simulink model "Reloadable_FIR"  (R2020a)
settings: Solver=VariableStepDiscrete  StartTime=0.0  StopTime=60  MaxStep=1  RelTol=1e-3  EnableMultiTasking=on
libraries: xbsIndex_r4 x15, dspsrcs4 x3, xbsCopyrightNotice_r4 x1
settings Model: Creator=arvinds  LastModifiedBy=viswanad
settings DataIOCC: LimitDataPoints=on  SaveFormat=Array  SignalLoggingSaveFormat=ModelDataLogs  ReturnWorkspaceOutputs=off
settings OptimizationCC: DefaultParameterBehavior=Inlined  ExpressionDepthLimit=2147483647  InitFltsAndDblsToZero=on  LifeSpan=inf
settings DebuggingCC: SaveWithParameterizedLinksMsg=none  UnderspecifiedInitializationDetection=Classic  MergeDetectMultiDrivingBlocksExec=none  SignalResolutionControl=TryResolveAllWithWarning  SolverPrmCheckMsg=warning  MultiTaskDSMMsg=warning  MultiTaskCondExecSysMsg=none  FcnCallInpInsideContextMsg=warning  AllowSymbolicDim=off  StateNameClashWarn=warning  SFUnexpectedBacktrackingDiag=warning  SFNoUnconditionalDefaultTransitionDiag=warning  SFExecutionAtInitializationDiag=none  ArithmeticOperatorsInVariantConditions=warning
settings HardwareCC: ProdBitPerPointer=32  ProdBitPerSizeT=32  ProdBitPerPtrDiffT=32  ProdLargestAtomicFloat=None  ProdIntDivRoundTo=Undefined  ProdEndianess=Unspecified  ProdWordSize=32  ProdHWDeviceType=32-bit Generic
settings ModelReferenceCC: PropagateSignalLabelsOutOfModel=off
settings SFSimCC: SimUseLocalCustomCode=off  CustomCodeUndefinedFunction=UseInterfaceOnly
settings RTWCC: RTWUseLocalCustomCode=off
settings CodeAppCC: StateflowObjectComments=on
settings GRTTargetCC: TargetFcnLib=ansi_tfl_tmw.mat  TargetLangStandard=C89/C90 (ANSI)  CombineOutputUpdateFcns=off  GRTInterface=on
settings ConfigComp: CovMetricSettings=dw  CovSaveCumulativeToWorkspaceVar=on  CovSaveSingleToWorkspaceVar=on  CovExternalEMLEnable=off

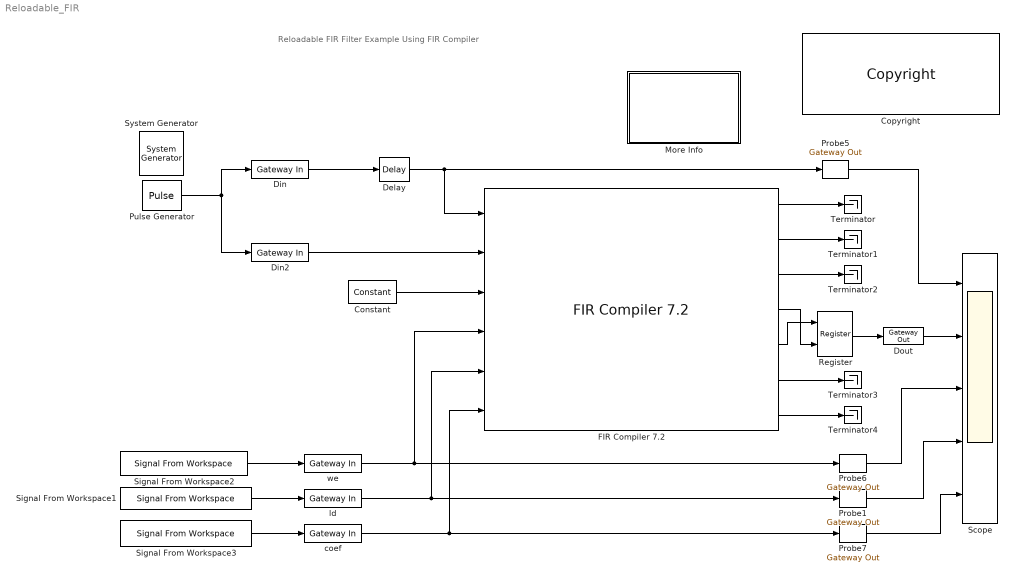
== system Reloadable_FIR ==
  note: Reloadable FIR Filter Example Using FIR Compiler
  " System Generator" : xbsIndex_r4/ System Generator  Tag=genX  xilinxfamily=kintex7  part=xc7k325t  speed=-3  package=fbg676  synthesis_tool=Vivado  clock_wrapper=Clock Enables  directory=./netlist  proj_type=Vivado  Synth_file=Vivado Synthesis Defaults  Impl_file=Vivado Implementation Defaults  testbench=off  simulink_period=1  sysclk_period=10  dcm_input_clock_period=10  incr_netlist=off  trim_vbits=Everywhere in SubSystem  dbl_ovrd=According to Block Masks  core_generation=According to Block Masks  run_coregen=off  deprecated_control=off  eval_field=0  block_type=sysgen
  Constant : xbsIndex_r4/Constant  const=0  gui_display_data_type=Fixed-point  arith_type=Unsigned  n_bits=8  bin_pt=0  preci_type=Single  exp_width=8  frac_width=24  explicit_period=off  period=1  equ=P=C  opselect=C  inp2=PCIN>>17  opr=+  inp1=P  carry=CIN  dbl_ovrd=off  block_type=constant
  Copyright : xbsCopyrightNotice_r4/Copyright  copyrighttext="Copyright (c) 2021  by  Xilinx, Inc. All rights reserved.<br><br>This file contains proprietary, confidential information of Xilinx, Inc., is distributed under license from Xilinx, Inc., and may be used, copied and/or disclosed only pursuant to the terms of a valid license agreement with Xilinx, Inc. Xilinx hereby grants you a license to use this file solely for design, simulation, implementation and creation of design files limited to Xilinx devices or technologies. Use with non-Xilinx devices or technologies is expressly prohibited and immediately terminates your license unless covered by a separate agreement.<br><br>Xilinx is providing this design, code, or information \"as-is\" solely for use in developing programs and solutions for Xilinx devices, with no obligation on the part of Xilinx to provide support. By providing this design, code, or information as one possible implementation of this feature, application or standard, Xilinx is making no representation that this implementation is free from any claims of infringement. You are responsible for obtaining any rights you may require for your implementation. Xilinx expressly disclaims any warranty whatsoever with respect to the adequacy of the implementation, including but not limited to any warranties or representations that this implementation is free from claims of infringement, implied warranties of merchantability or fitness for a particular purpose.<br><br>Xilinx products are not intended for use in life support appliances, devices, or systems. Use in such applications is expressly prohibited.<br><br>Any modifications that are made to the Source Code are done at the user's sole risk and will be unsupported.<br><br>This copyright and support notice must be retained as part of this text at all times. (c) Copyright 1995-2021 Xilinx, Inc. All rights reserved."  block_type=copyright
  Delay : xbsIndex_r4/Delay  rst=off  infoeditControl=Selection of Reset will increase slice count due to use of real FFs and instead of SRLs  en=off  latency=1  reg_retiming=off  dbl_ovrd=off  block_type=delay
  Din : xbsIndex_r4/Gateway In  gui_display_data_type=Fixed-point  arith_type="Signed  (2's comp)"  n_bits=16  bin_pt=0  preci_type=Single  exp_width=8  frac_width=24  rows=1  columns=1  quantization="Round  (unbiased: +/- Inf)"  overflow=Saturate  period=1  UseAsADC=off  ADCChannel='1'  interface=None  automatic_assignment=on  address_offset=hex2dec('00')  intf_name=''  intf_description=''  default_value=0  timing_constraint=None  locs_specified=off  LOCs={}  io_standard={}  inherit_from_input=off  hdl_port=on  dbl_ovrd=off  block_type=gatewayin
  Din2 : xbsIndex_r4/Gateway In  gui_display_data_type=Boolean  arith_type=Boolean  n_bits=8  bin_pt=0  preci_type=Single  exp_width=8  frac_width=24  rows=1  columns=1  quantization="Round  (unbiased: +/- Inf)"  overflow=Saturate  period=1  UseAsADC=off  ADCChannel='1'  interface=None  automatic_assignment=on  address_offset=hex2dec('00')  intf_name=''  intf_description=''  default_value=0  timing_constraint=None  locs_specified=off  LOCs={}  io_standard={}  inherit_from_input=off  hdl_port=on  dbl_ovrd=off  block_type=gatewayin
  Dout : xbsIndex_r4/Gateway Out  inherit_from_input=off  hdl_port=on  rows=1  columns=1  UseAsDAC=off  DACChannel='1'  interface=None  automatic_assignment=on  address_offset=hex2dec('00')  intf_name=''  intf_description=''  timing_constraint=None  locs_specified=off  LOCs={}  io_standard={}  block_type=gatewayout
  FIR Compiler 7.2 : xbsIndex_r4/FIR Compiler 7.2   coefficientvector=[1,2,3,2,1]  coefficient_sets=1  coefficient_reload=on  filter_type=Single_Rate  rate_change_type=Integer  interpolation_rate=1  decimation_rate=1  zero_pack_factor=1  channel_sequence=Basic  number_channels=1  pattern_list='P4-0,P4-1,P4-2,P4-3,P4-4'  number_paths=1  ratespecification=Maximum_Possible  sampleperiod=1  hardwareoversamplingrate=1  coefficient_sign=Signed  quantization=Integer_Coefficients  coefficient_width=16  bestprecision=off  coefficient_fractional_bits=0  coefficient_structure=Inferred  output_rounding_mode=Full_Precision  output_width=35  filter_architecture=Systolic_Multiply_Accumulate  optimization_goal=Area  optimization_list='None'  data_buffer_type=Automatic  coefficient_buffer_type=Automatic  input_buffer_type=Automatic  output_buffer_type=Automatic  preference_for_other_storage=Automatic  multi_column_support=Automatic  columnconfig='5'  inter_column_pipe_length=4  data_has_tlast=Not_Required  m_data_has_tready=off  s_data_has_fifo=off  s_data_has_tuser=Not_Required  m_data_has_tuser=Not_Required  s_config_sync_mode=On_Vector  s_config_method=Single  num_reload_slots=1  has_aclken=off  has_aresetn=off  infoeditControl=ARESETn must be asserted for a minimum of 2 cycles  reset_data_vector=on  trim_axipin_name=on  simulation_type=hybrid_sim  simulation_model=sysgen:xfirv7_2_cmodel  data_path_portlist={ 's_axis_data_tdata', 'm_axis_data_tdata' }  passband_min=0.0  passband_max=0.5  stopband_min=0.5  stopband_max=1.0  filter_selection=1  gui_behaviour='Sysgen_GUI'  data_sign=Signed  data_width=16  data_fractional_bits=0  data_tuser_width=1  wrapper_available=true  ip_wrap_arbitrary_binary_point=true  ip_name=FIR Compiler  ip_version=7.2  dsptool_ready=true  ipcore_usecache=true  ipcore_useipmodelcache=true  port_translation_map={ 'aclken' => 'en', 'aresetn' => 'rst' }  run_core_at_system_period=true  ipcore_xco_need_fpga_part=true  block_type=fir_compiler_v7_2
      settings: infoedit=Maximum Possible : Maximizes oversampling rate. Abstracted input handshake (no s_data_tvalid) and automatic rate propagation.<br>Hardware Oversampling Rate : Specifies oversampling rate relative to the input sample period. Abstracted input handshake (no s_data_tvalid) and automatic rate propagation.<br>Input/Output Sample Period : Specifies absolute oversampling rate. No input handshake abstraction (exposes s_data_tvalid) and no rate propagation.
  More Info : Subsystem
      mask Display: disp('Double click\n for\n more information.')
  Probe{1,5..7} (4 alike) : xbsIndex_r4/Gateway Out  inherit_from_input=off  hdl_port=off  rows=1  columns=1  UseAsDAC=off  DACChannel='1'  interface=None  automatic_assignment=on  address_offset=hex2dec('00')  intf_name=''  intf_description=''  timing_constraint=None  locs_specified=off  LOCs={}  io_standard={}  block_type=gatewayout
  Pulse Generator : DiscretePulseGenerator  Period=30  VectorParams1D=off
  Register : xbsIndex_r4/Register  init=0  rst=off  en=on  dbl_ovrd=off  block_type=register
  Scope : Scope  NumInputPorts=5
  Signal From Workspace1 : dspsrcs4/Signal From Workspace  X=[ zeros(1,19) 1 0]  Ts=1  nsamps=1  OutputAfterFinalValue=Setting to zero  ignoreOrWarnInputAndFrameLengths=off  OutputFrames=on
  Signal From Workspace2 : dspsrcs4/Signal From Workspace  X=[ zeros(1,20) 1 1 1 0]  Ts=1  nsamps=1  OutputAfterFinalValue=Setting to zero  ignoreOrWarnInputAndFrameLengths=off  OutputFrames=on
  Signal From Workspace3 : dspsrcs4/Signal From Workspace  X="[ zeros(1,20)  7 8 9 0]"  Ts=1  nsamps=1  OutputAfterFinalValue=Setting to zero  ignoreOrWarnInputAndFrameLengths=off  OutputFrames=on
  Terminator{,1..4} (5 alike) : Terminator
  coef : xbsIndex_r4/Gateway In  gui_display_data_type=Fixed-point  arith_type=Unsigned  n_bits=16  bin_pt=0  preci_type=Single  exp_width=8  frac_width=24  rows=1  columns=1  quantization="Round  (unbiased: +/- Inf)"  overflow=Saturate  period=1  UseAsADC=off  ADCChannel='1'  interface=None  automatic_assignment=on  address_offset=hex2dec('00')  intf_name=''  intf_description=''  default_value=0  timing_constraint=None  locs_specified=off  LOCs={}  io_standard={}  inherit_from_input=off  hdl_port=on  dbl_ovrd=off  block_type=gatewayin
  ld : xbsIndex_r4/Gateway In  gui_display_data_type=Boolean  arith_type=Boolean  n_bits=16  bin_pt=8  preci_type=Single  exp_width=8  frac_width=24  rows=1  columns=1  quantization="Round  (unbiased: +/- Inf)"  overflow=Saturate  period=1  UseAsADC=off  ADCChannel='1'  interface=None  automatic_assignment=on  address_offset=hex2dec('00')  intf_name=''  intf_description=''  default_value=0  timing_constraint=None  locs_specified=off  LOCs={}  io_standard={}  inherit_from_input=off  hdl_port=on  dbl_ovrd=off  block_type=gatewayin
  we : xbsIndex_r4/Gateway In  gui_display_data_type=Boolean  arith_type=Boolean  n_bits=16  bin_pt=8  preci_type=Single  exp_width=8  frac_width=24  rows=1  columns=1  quantization="Round  (unbiased: +/- Inf)"  overflow=Saturate  period=1  UseAsADC=off  ADCChannel='1'  interface=None  automatic_assignment=on  address_offset=hex2dec('00')  intf_name=''  intf_description=''  default_value=0  timing_constraint=None  locs_specified=off  LOCs={}  io_standard={}  inherit_from_input=off  hdl_port=on  dbl_ovrd=off  block_type=gatewayin
  wires:
  Din/1 -> Delay/1
  Pulse Generator/1 -> Din/1, Din2/1
  Signal From Workspace1/1 -> ld/1
  ld/1 -> Probe1/1, FIR Compiler 7.2/5
  Signal From Workspace2/1 -> we/1
  we/1 -> Probe6/1, FIR Compiler 7.2/4
  Signal From Workspace3/1 -> coef/1
  coef/1 -> Probe7/1, FIR Compiler 7.2/6
  Register/1 -> Dout/1
  Probe5/1 -> Scope/1
  Probe6/1 -> Scope/3
  Probe7/1 -> Scope/5
  Delay/1 -> Probe5/1, FIR Compiler 7.2/1
  Dout/1 -> Scope/2
  Probe1/1 -> Scope/4
  Constant/1 -> FIR Compiler 7.2/3
  Din2/1 -> FIR Compiler 7.2/2
  FIR Compiler 7.2/5 -> Register/1
  FIR Compiler 7.2/1 -> Terminator/1
  FIR Compiler 7.2/2 -> Terminator1/1
  FIR Compiler 7.2/3 -> Terminator2/1
  FIR Compiler 7.2/6 -> Terminator3/1
  FIR Compiler 7.2/7 -> Terminator4/1
  FIR Compiler 7.2/4 -> Register/2

== system Reloadable_FIR/More Info ==
  note: Reloadable FIR Filter Example Using FIR Compiler
  note: This design example shows how the FIR Compiler block can be configured as a reloadable coefficient FIR filter.
      | The first set of coefficients is specified and loaded by the core, and the second set is loaded from an external
      | source using the xlGetReOrderedCoeff function below. This function is needed in the sequence of events to
      | reload new filter coefficients.
      |
      | A = xlGetReOrderedCoeff(new_coeff_set, returnType, block_handle)
      |
      | where
      |
      | new_coeff_set  =  New coefficient set to be loaded
      | returnType        =  Coeff or Index
      | block_handle    =  FIR Compiler block handle in the design which can be specified as 'gcbh'
      |
      | To understand the use and advantages of this function in the FIR Compiler 7.2 System Generator design,
      | observe the following:
      |
      | •	Double-click the FIR Compiler block and you can see the set of coefficients [1 2 3 2 1] was specified.
      |      This set of coefficients is pre-loaded in the core.
      |
      | •	The set of inputs connected to the FIR Compiler block (reload_tvalid, reload_tlast, and
      |       reload_tdata_data) perform the following on the FIR Compiler 7.2 block:
      | 	•	reload_tdata_data and reload_tvalid: After the initial set of coefficients specified  by the core [1 2 3 2 1]
      |             is compiled, the new set of coefficients ([7 8 9 0]) is loaded via the reload_tdata_data input port.
      |             The reload _tvalid control signal must be high during this reload period. In this case reload _tvalid must
      |             be high for 3 clock cycles.
      |             In the Scope block, the reload_tdata_data signal appears as coef_din, and the reload _tvalid signal
      |             appears as coef_we.
      | 	•	reload_tlast: This signal must be high on the last coefficient data to indicate that the last data has been
      |             loaded. In the Scope block, the reload_tlast signal appears as coef_ld.
      |
      | •	The inputs that are connected to the three reload_* signals are vectors in this format:
      | 	•	reload_tvalid has input [zeros(1,20) 1 1 1 0]  = [0 0 0 0 0 0 0 0 0 0 0 0 0 0 0 0 0 0 0 0 0 1 1 1 0].
      | 	      The format zeros(1,N) returns 1-by-N vectors of zeros. This is “zero padding”, an interpolation method
      | 		which interprets time-domain samples as extending from 0 to N-1.
      | 	•	reload_tlast has input [zeros(1,19 1 0]. reload_tlast goes high at the 20th simulation time for 1 sample
      | 		period to indicate the last coefficient data.
      | 	•	Similarly, reload_tdata_data has input as [zeros(1,20) 7 8 9].
      |
      | 	Now, Double-click the Scope block and observe the following:
      |
      | 	•	The reload _tvalid control signal (coef_we in the Scope display) goes high during the reload period,
      | 		when the new set of coefficients is loaded via the reload_tdata_data input port (coef_din in the Scope
      |             display).
      |             coef_we goes high after the 20th simulation time for 3 clock cycles.
      | 	•	reload_tlast (coef_ld in the Scope display) goes high at the 20th simulation time for 1 sample period,
      | 		to indicate the last coefficient data.
      |
      |
      | Coefficients can be symmetric or asymmetric.
      |
      | Example :
      |
      | 1.	In the Simulink model, select the FIR Compiler 7.2 block.
      |
      | 2.	In the MATLAB Command Window, enter the following commands:
      |
      | 		>new_coeff = [7 8 9 0 9]
      |
      | 		 new_coeff =
      |
      | 		     7     8     9     0   9
      |
      | 		>xlGetReOrderedCoeff(new_coeff,'coeff',gcbh)
      |
      | 		ans =
      |
      | 		     7
      |  		     8
      | 		     9
